simulink model "Non_Linear_Simulator_B747"  (R2020a)
settings: Solver=ode4  StartTime=0.0  StopTime=200  FixedStep=0.01  RelTol=1e-3
libraries: simulink_extras x7, shared6dof x1, vrlib x1
settings Model: OrderedModelArguments=off  Creator=mohan  LastModifiedBy=mohan

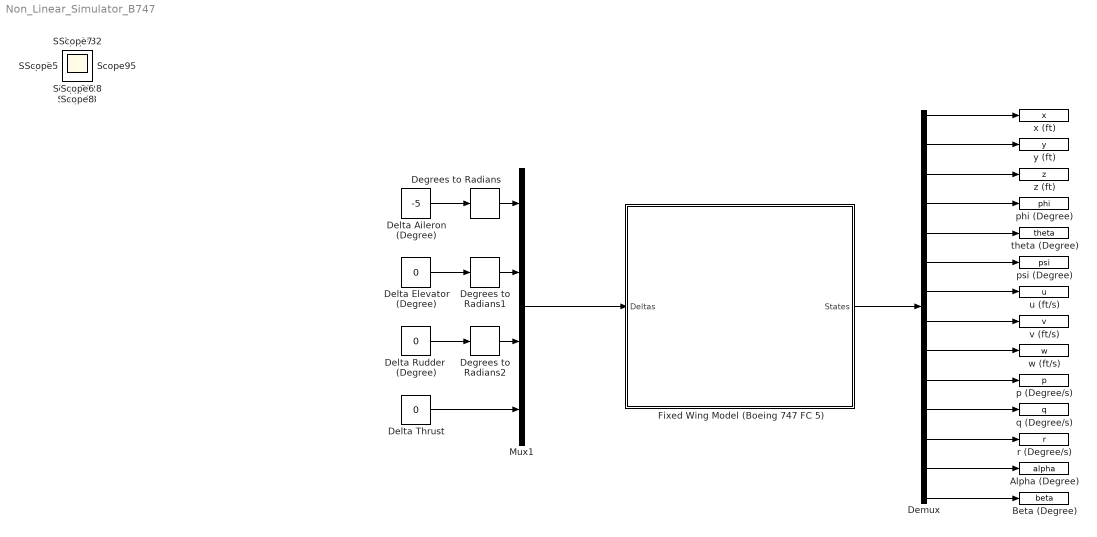
== system Non_Linear_Simulator_B747 ==
  Alpha (Degree) : ToWorkspace  VariableName=alpha  SaveFormat=Timeseries  SampleTime=-1
  Beta (Degree) : ToWorkspace  VariableName=beta  SaveFormat=Timeseries  SampleTime=-1
  Degrees to Radians : simulink_extras/Transformations/Degrees to Radians
  Degrees to Radians1 : simulink_extras/Transformations/Degrees to Radians
  Degrees to Radians2 : simulink_extras/Transformations/Degrees to Radians
  Delta Aileron (Degree) : Constant  Value=-5
  Delta Elevator (Degree) : Constant  Value=0
  Delta Rudder  (Degree) : Constant  Value=0
  Delta Thrust : Constant  Value=0
  Demux : Demux  Outputs=14
  Fixed Wing Model (Boeing 747 FC 5) : Subsystem  mask{m=19787.25091, g=32.17405, Ixx=1.82E+07, Iyy=3.31E+07, Izz=4.97E+07, Ixz=9.70E+05, Ixy=0, Iyz=0, L_th=1, VT=518, t0=0, tf=200, h=0.01, Xu=-0.00247, Zu=-0.0679, Mu=0.000247, Xw=0.0782, Zw=-0.433, Mw=-0.00170, Zw_dot=0.0157, Zq=-6.39, Mw_dot=-0.000125, Mq=-0.0421, Xdel_e=2.02, Zdel_e=-16.9, Mdel_e=-1.09, Xdel_t=0.505e-4, Zdel_t=-0.220e-5, Mdel_t=0.302e-6, Yv=-0.0822, YB=-42.6, LB_dash=-2.05, NB_dash=0.419, Lp_dash=-0.652, Np_dash=-0.0701, Lr_dash=0.376, Nr_dash=-0.140, Ydel_a_star=0, Ldel_a_dash=0.128, Ndel_a_dash=0.0177, Ydel_r_star=0.0131, Ldel_r_dash=0.148, Ndel_r_dash=-0.381, Yp=0, Yr=0, x0=0, y0=0, z0=-20000, u_0=514.3561332, v_0=0, w_0=61.33325558, p_0=0, q_0=0, r_0=0, udot_0=0, vdot_0=0, wdot_0=0, phai_0=0, theta_0=6.8*pi/180, psi_0=0}
      mask prompts: m "Mass"; g "Gravity"; L_th "Perpindicular Distance to Thrust Line from C.G"; VT "True Speed (FPS)"; t0 "Start Time"; tf "Stop Time"; h "Time Step"
      mask DialogControl Time Prompt: Time Properties
      mask DialogControl Derivatives Prompt: Aerodynamics Derivatives
      mask DialogControl States Prompt: Initial States
      mask Display: image('$imagefile'); % Use "Edit Image" on toolstrip to change.
  Mux1 : Mux
  p (Degree/s) : ToWorkspace  VariableName=p  SaveFormat=Timeseries  SampleTime=-1
  phi (Degree) : ToWorkspace  VariableName=phi  SaveFormat=Timeseries  SampleTime=-1
  psi (Degree) : ToWorkspace  VariableName=psi  SaveFormat=Timeseries  SampleTime=-1
  q (Degree/s) : ToWorkspace  VariableName=q  SaveFormat=Timeseries  SampleTime=-1
  r (Degree/s) : ToWorkspace  VariableName=r  SaveFormat=Timeseries  SampleTime=-1
  theta (Degree) : ToWorkspace  VariableName=theta  SaveFormat=Timeseries  SampleTime=-1
  u (ft/s) : ToWorkspace  VariableName=u  SaveFormat=Timeseries  SampleTime=-1
  v (ft/s) : ToWorkspace  VariableName=v  SaveFormat=Timeseries  SampleTime=-1
  w (ft/s) : ToWorkspace  VariableName=w  SaveFormat=Timeseries  SampleTime=-1
  x (ft) : ToWorkspace  VariableName=x  SaveFormat=Timeseries  SampleTime=-1
  y (ft) : ToWorkspace  VariableName=y  SaveFormat=Timeseries  SampleTime=-1
  z (ft) : ToWorkspace  VariableName=z  SaveFormat=Timeseries  SampleTime=-1
  Scope{,1..33} (34 alike) : Scope
  wires:
  Delta Elevator (Degree)/1 -> Degrees to Radians1/1
  Delta Thrust/1 -> Mux1/4
  Delta Aileron (Degree)/1 -> Degrees to Radians/1
  Delta Rudder  (Degree)/1 -> Degrees to Radians2/1
  Mux1/1 -> Fixed Wing Model (Boeing 747 FC 5)/1(Deltas)
  Fixed Wing Model (Boeing 747 FC 5)/1(States) -> Demux/1
  Demux/1 -> x (ft)/1
  Demux/2 -> y (ft)/1
  Demux/3 -> z (ft)/1
  Demux/5 -> theta (Degree)/1
  Demux/7 -> u (ft/s)/1
  Demux/8 -> v (ft/s)/1
  Demux/9 -> w (ft/s)/1
  Demux/10 -> p (Degree/s)/1
  Demux/11 -> q (Degree/s)/1
  Demux/12 -> r (Degree/s)/1
  Demux/13 -> Alpha (Degree)/1
  Demux/14 -> Beta (Degree)/1
  Degrees to Radians/1 -> Mux1/1
  Degrees to Radians1/1 -> Mux1/2
  Degrees to Radians2/1 -> Mux1/3
  Demux/4 -> phi (Degree)/1
  Demux/6 -> psi (Degree)/1

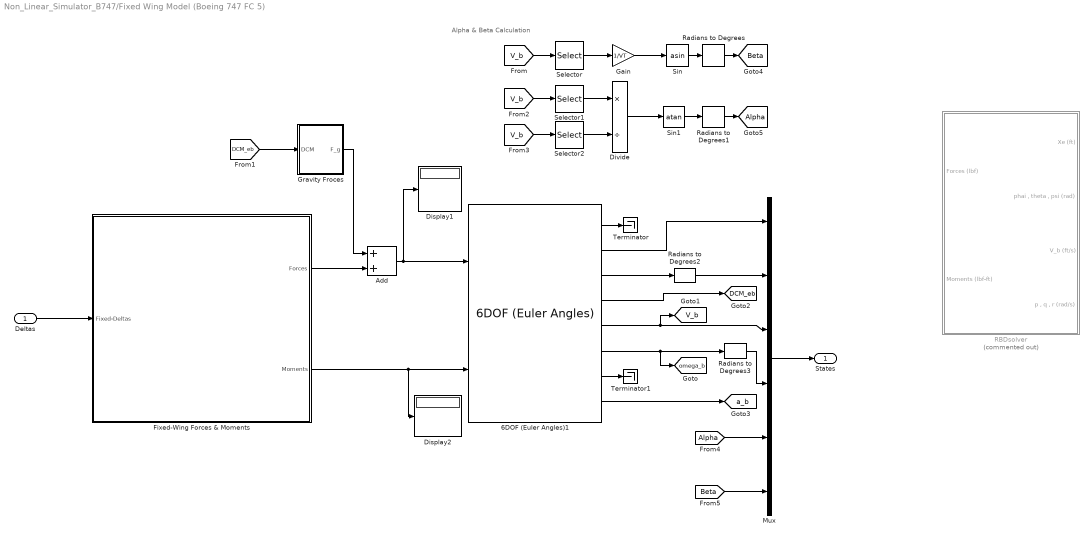
== system Non_Linear_Simulator_B747/Fixed Wing Model (Boeing 747 FC 5) ==
  note: Alpha & Beta Calculation
  Deltas : Inport
  6DOF (Euler Angles)1 : shared6dof/6DOF (Euler Angles)  units=English (Velocity in ft/s)  mtype=Fixed  rep=Euler Angles  xme_0=[x0 y0 z0]  Vm_0=[u_0 v_0 w_0]  eul_0=[phai_0 theta_0 psi_0]  pm_0=[p_0 q_0 r_0]  mass_0=m  mass_e=0.5  mass_f=2.0  inertia=[Ixx -Ixy -Ixz ; -Ixy Iyy -Iyz ; -Ixz -Iyz Izz]  inertia_e=eye(3)  inertia_f=2*eye(3)  k_quat=1.0  vre_flag=on  abi_flag=off  aMode=aMode  xme_statename=''  Vm_statename=''  eul_statename=''  quat_statename=''  pm_statename=''  mass_statename=''
      settings: SourceProductBaseCode=AE,PW,MT,VE,VP
  Add : Sum  Inputs=2
  Display1 : Display
  Display2 : Display
  Divide : Product  Inputs=*/
  Fixed-Wing Forces & Moments : Subsystem
  Gain : Gain  Gain=1/VT
  Gravity Froces : Subsystem
  Mux : Mux  Inputs=6
  RBDsolver : Subsystem  Commented=on
  Radians to Degrees{,1..3} (4 alike) : simulink_extras/Transformations/Radians to Degrees
  Selector : Selector  InputPortWidth=3  IndexOptions=Starting index (dialog)  Indices=2  OutputSizes=1
  Selector1 : Selector  InputPortWidth=3  IndexOptions=Starting index (dialog)  Indices=3  OutputSizes=1
  Selector2 : Selector  InputPortWidth=3  IndexOptions=Starting index (dialog)  Indices=1  OutputSizes=1
  Sin : Trigonometry  Operator=asin
  Sin1 : Trigonometry  Operator=atan
  Terminator : Terminator
  Terminator1 : Terminator
  States : Outport
  tag scope: Alpha=global, Beta=global, DCM_eb=global, V_b=global, a_b=global, omega_b=global
  wires:
  Gravity Froces/1(F_g) -> Add/1
  6DOF (Euler Angles)1/2 -> Mux/1
  6DOF (Euler Angles)1/1 -> Terminator/1
  Mux/1 -> States/1
  6DOF (Euler Angles)1/7 -> Terminator1/1
  Fixed-Wing Forces & Moments/1(Forces) -> Add/2
  Add/1 -> 6DOF (Euler Angles)1/1, Display1/1
  Fixed-Wing Forces & Moments/2("Moments ") -> Display2/1, 6DOF (Euler Angles)1/2
  6DOF (Euler Angles)1/4 -> [DCM_eb]
  6DOF (Euler Angles)1/8 -> [a_b]
  [DCM_eb] -> Gravity Froces/1(DCM)
  [V_b] -> Selector/1
  Selector/1 -> Gain/1
  Gain/1 -> Sin/1
  Sin/1 -> Radians to Degrees/1
  Divide/1 -> Sin1/1
  Selector1/1 -> Divide/1
  Sin1/1 -> Radians to Degrees1/1
  [V_b] -> Selector1/1
  [V_b] -> Selector2/1
  Selector2/1 -> Divide/2
  [Alpha] -> Mux/5
  [Beta] -> Mux/6
  Radians to Degrees/1 -> [Beta]
  Radians to Degrees1/1 -> [Alpha]
  6DOF (Euler Angles)1/3 -> Radians to Degrees2/1
  6DOF (Euler Angles)1/6 -> [omega_b], Radians to Degrees3/1
  Deltas/1 -> Fixed-Wing Forces & Moments/1(Fixed-Deltas)
  Radians to Degrees2/1 -> Mux/2
  6DOF (Euler Angles)1/5 -> Mux/3, [V_b]
  Radians to Degrees3/1 -> Mux/4

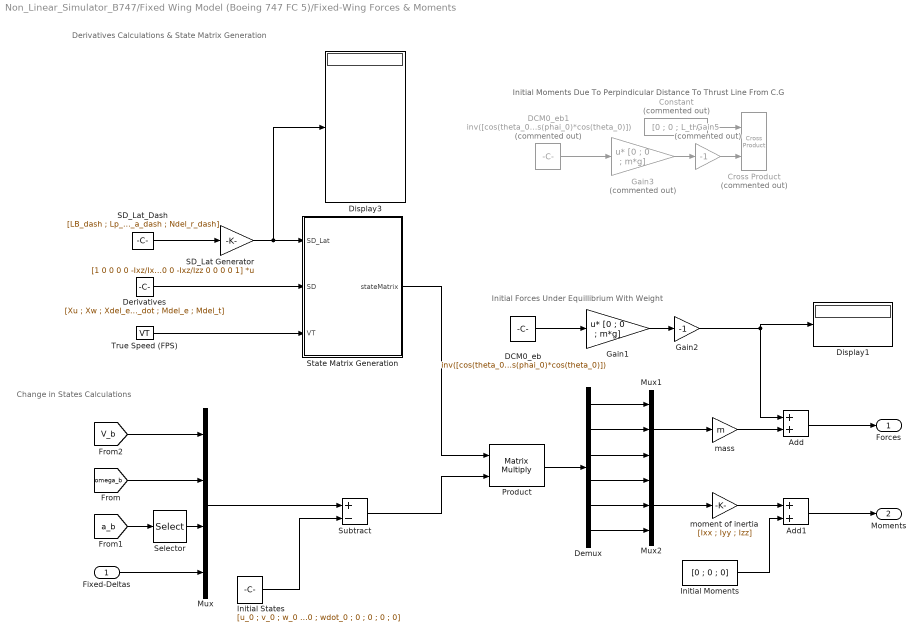
== system Non_Linear_Simulator_B747/Fixed Wing Model (Boeing 747 FC 5)/Fixed-Wing Forces & Moments ==
  note: Change in States Calculations
  note: Derivatives Calculations & State Matrix Generation
  note: Initial Forces Under Equillibrium With Weight
  note: Initial Moments Due To Perpindicular Distance To Thrust Line From C.G
  Fixed-Deltas : Inport
  Add : Sum
  Add1 : Sum
  Constant : Constant  Commented=on  Value=[0 ; 0 ; L_th]
  Cross Product : vrlib/Utilities/Cross Product  Commented=on
  DCM0_eb : Constant  Value="inv([cos(theta_0)*cos(psi_0) , (sin(phai_0)*sin(theta_0)*cos(psi_0)-cos(phai_0)*sin(psi_0)) , (cos(phai_0)*sin(theta_0)*cos(psi_0)+sin(phai_0)*sin(psi_0)) ; cos(theta_0)*sin(psi_0) , (sin(phai_0)*sin(theta_0)*sin(psi_0)+cos(phai_0)*cos(psi_0)) , (cos(phai_0)*sin(theta_0)*sin(psi_0)-sin(phai_0)*cos(psi_0)) ;  -sin(theta_0) ,  sin(phai_0)*cos(theta_0)  , cos(phai_0)*cos(theta_0)])"
  DCM0_eb1 : Constant  Commented=on  Value="inv([cos(theta_0)*cos(psi_0) , (sin(phai_0)*sin(theta_0)*cos(psi_0)-cos(phai_0)*sin(psi_0)) , (cos(phai_0)*sin(theta_0)*cos(psi_0)+sin(phai_0)*sin(psi_0)) ; cos(theta_0)*sin(psi_0) , (sin(phai_0)*sin(theta_0)*sin(psi_0)+cos(phai_0)*cos(psi_0)) , (cos(phai_0)*sin(theta_0)*sin(psi_0)-sin(phai_0)*cos(psi_0)) ;  -sin(theta_0) ,  sin(phai_0)*cos(theta_0)  , cos(phai_0)*cos(theta_0)])"
  Demux : Demux  Outputs=6
  Derivatives : Constant  Value=[Xu ; Xw ; Xdel_e ; Xdel_t ; Yv ; Yp ; Yr ; Ydel_r_star ; Zu ; Zw ; Zq ; Zw_dot ; Zdel_e ; Zdel_t ; Mu ; Mw ; Mq ; Mw_dot ; Mdel_e ; Mdel_t]
  Display1 : Display
      settings: Decimation=4
  Display3 : Display
  Gain1 : Gain  Gain=[0 ; 0 ; m*g]  Multiplication=Matrix(u*K)
  Gain2 : Gain  Gain=-1
  Gain3 : Gain  Commented=on  Gain=[0 ; 0 ; m*g]  Multiplication=Matrix(u*K)
  Gain5 : Gain  Commented=on  Gain=-1
  Initial Moments : Constant  Value=[0 ; 0 ; 0]
  Initial States : Constant  Value=[u_0 ; v_0 ; w_0 ; p_0 ; q_0 ; r_0 ; wdot_0 ; 0 ; 0 ; 0 ; 0]
  Mux : Mux
  Mux1 : Mux  Inputs=3
  Mux2 : Mux  Inputs=3
  Product : Product  Multiplication=Matrix(*)
  SD_Lat Generator : Gain  Gain="[1 0 0 0 0 -Ixz/Ixx 0 0 0 0 ; 0 1 0 0 0 0 -Ixz/Ixx 0 0 0 ; 0 0 1 0 0 0 0 -Ixz/Ixx 0  0 ; 0 0 0 1 0 0 0 0 -Ixz/Ixx 0 ; 0 0 0 0 1 0 0 0 0 -Ixz/Ixx ; -Ixz/Izz 0 0 0 0 1 0 0 0 0 ; 0 -Ixz/Izz 0 0 0 0 1 0 0 0 ; 0 0 -Ixz/Izz 0 0 0 0 1 0 0 ; 0 0 0 -Ixz/Izz 0 0 0 0 1 0 ;  0 0 0 0 -Ixz/Izz 0 0 0 0 1]"  Multiplication=Matrix(K*u)
  SD_Lat_Dash : Constant  Value=[LB_dash ; Lp_dash ; Lr_dash ; Ldel_a_dash ; Ldel_r_dash ; NB_dash ; Np_dash ; Nr_dash ; Ndel_a_dash ; Ndel_r_dash]
  Selector : Selector  InputPortWidth=3  IndexOptions=Starting index (dialog)  Indices=3  OutputSizes=1
  State Matrix Generation : MATLAB Function  TreatAsAtomicUnit=on
  Subtract : Sum  Inputs=+-
  True Speed (FPS) : Constant  Value=VT
  mass : Gain  Gain=m
  moment of inertia : Gain  Gain=[Ixx ; Iyy ; Izz]
  Forces : Outport
  "Moments " : Outport  Port=2
  wires:
  Selector/1 -> Mux/3
  Fixed-Deltas/1 -> Mux/4
  [omega_b] -> Mux/2
  [V_b] -> Mux/1
  Mux/1 -> Subtract/1
  Subtract/1 -> Product/2
  Initial States/1 -> Subtract/2
  Demux/2 -> Mux1/2
  Demux/1 -> Mux1/1
  Demux/3 -> Mux1/3
  Demux/4 -> Mux2/1
  Demux/5 -> Mux2/2
  Demux/6 -> Mux2/3
  Mux1/1 -> mass/1
  Mux2/1 -> moment of inertia/1
  mass/1 -> Add/2
  moment of inertia/1 -> Add1/1
  Add/1 -> Forces/1
  Add1/1 -> "Moments "/1
  DCM0_eb/1 -> Gain1/1
  Gain1/1 -> Gain2/1
  Gain2/1 -> Add/1, Display1/1
  Gain3/1 -> Gain5/1
  DCM0_eb1/1 -> Gain3/1
  Gain5/1 -> Cross Product/2
  Constant/1 -> Cross Product/1
  Initial Moments/1 -> Add1/2
  SD_Lat_Dash/1 -> SD_Lat Generator/1
  SD_Lat Generator/1 -> Display3/1, State Matrix Generation/1(SD_Lat)
  Product/1 -> Demux/1
  State Matrix Generation/1(stateMatrix) -> Product/1
  Derivatives/1 -> State Matrix Generation/2(SD)
  True Speed (FPS)/1 -> State Matrix Generation/3(VT)
  [a_b] -> Selector/1

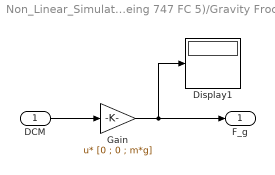
== system Non_Linear_Simulator_B747/Fixed Wing Model (Boeing 747 FC 5)/Gravity Froces ==
  DCM : Inport
  Display1 : Display
  Gain : Gain  Gain=[0 ; 0 ; m*g]  Multiplication=Matrix(u*K)
  F_g : Outport
  wires:
  Gain/1 -> F_g/1, Display1/1
  DCM/1 -> Gain/1

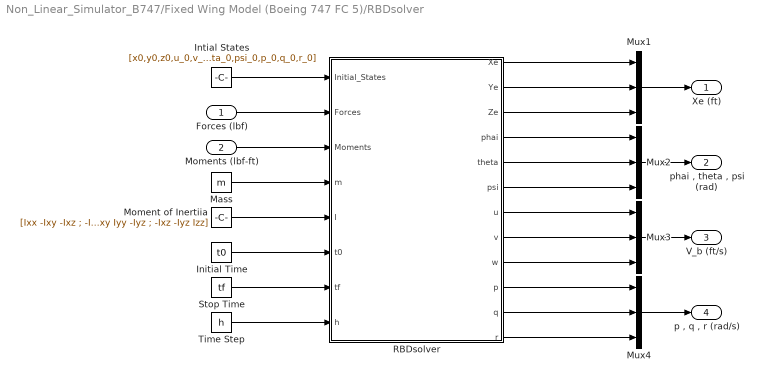
== system Non_Linear_Simulator_B747/Fixed Wing Model (Boeing 747 FC 5)/RBDsolver ==
  Forces (lbf) : Inport
  Moments (lbf-ft) : Inport  Port=2
  Initial Time : Constant  Value=t0
  Intial States : Constant  Value=[x0,y0,z0,u_0,v_0,w_0,phai_0,theta_0,psi_0,p_0,q_0,r_0]
  Mass : Constant  Value=m
  Moment of Inertiia : Constant  Value=[Ixx -Ixy -Ixz ; -Ixy Iyy -Iyz ; -Ixz -Iyz Izz]
  Mux{1..4} (4 alike) : Mux  Inputs=3
  RBDsolver : MATLAB Function  TreatAsAtomicUnit=on
  Stop Time : Constant  Value=tf
  Time Step : Constant  Value=h
  Xe (ft) : Outport
  "phai , theta , psi (rad)" : Outport  Port=2
  V_b (ft/s) : Outport  Port=3
  "p , q , r (rad/s)" : Outport  Port=4
  wires:
  RBDsolver/5(theta) -> Mux2/2
  Intial States/1 -> RBDsolver/1(Initial_States)
  Forces (lbf)/1 -> RBDsolver/2(Forces)
  RBDsolver/11(q) -> Mux4/2
  RBDsolver/7(u) -> Mux3/1
  RBDsolver/8(v) -> Mux3/2
  RBDsolver/9(w) -> Mux3/3
  Mass/1 -> RBDsolver/4(m)
  Moments (lbf-ft)/1 -> RBDsolver/3(Moments)
  Stop Time/1 -> RBDsolver/7(tf)
  Initial Time/1 -> RBDsolver/6(t0)
  RBDsolver/10(p) -> Mux4/1
  Time Step/1 -> RBDsolver/8(h)
  Moment of Inertiia/1 -> RBDsolver/5(I)
  RBDsolver/6(psi) -> Mux2/3
  RBDsolver/4(phai) -> Mux2/1
  RBDsolver/1(Xe) -> Mux1/1
  RBDsolver/3(Ze) -> Mux1/3
  RBDsolver/2(Ye) -> Mux1/2
  RBDsolver/12(r) -> Mux4/3
  Mux1/1 -> Xe (ft)/1
  Mux2/1 -> "phai , theta , psi (rad)"/1
  Mux3/1 -> V_b (ft/s)/1
  Mux4/1 -> "p , q , r (rad/s)"/1

== matlab function Non_Linear_Simulator_B747/Fixed Wing Model (Boeing 747 FC 5)/Fixed-Wing Forces & Moments/State Matrix Generation ==
  data: SD_Lat input; stateMatrix output; SD input; VT input
function stateMatrix = stateMatrixGenerator(SD_Lat,SD,VT)
stateMatrix=zeros(6,11);

Xu=SD(1);   Xw=SD(2);       Xdel_e=SD(3);       Xdel_t=SD(4);   Yv=SD(5);
Yp=SD(6);   Yr=SD(7);       Ydel_r_star=SD(8);  Zu=SD(9);       Zw=SD(10);
Zq=SD(11);  Zw_dot=SD(12);  Zdel_e=SD(13);      Zdel_t=SD(14);   Mu=SD(15); 
Mw=SD(16);  Mq=SD(17);      Mw_dot=SD(18);      Mdel_e=SD(19);   Mdel_t=SD(20);

LB=SD_Lat(1);   Lp=SD_Lat(2);   Lr=SD_Lat(3);   Ldel_a=SD_Lat(4);
Ldel_r=SD_Lat(5);
NB=SD_Lat(6);   Np=SD_Lat(7);   Nr=SD_Lat(8);   Ndel_a=SD_Lat(9);   
Ndel_r=SD_Lat(10);

Ydel_r=Ydel_r_star*VT;
Lv=LB/VT;
Nv=NB/VT;

stateMatrix=...
     [Xu , 0 , Xw , 0 , 0 , 0 , 0 , 0 , Xdel_e , 0 , Xdel_t ; 
      0 , Yv , 0 , Yp , 0 , Yr , 0 , 0 , 0 , Ydel_r , 0 ; 
      Zu , 0 , Zw , 0 , Zq , 0 , Zw_dot , 0 , Zdel_e , 0 , Zdel_t ; 
      0 , Lv , 0 , Lp , 0 , Lr , 0 , Ldel_a , 0 , Ldel_r , 0 ; 
      Mu , 0 , Mw , 0 , Mq , 0 , Mw_dot , 0 , Mdel_e , 0 , Mdel_t ; 
      0 , Nv , 0 , Np , 0 , Nr , 0 , Ndel_a , 0 , Ndel_r , 0];
end

== matlab function Non_Linear_Simulator_B747/Fixed Wing Model (Boeing 747 FC 5)/RBDsolver/RBDsolver ==
  data: Initial_States input; Xe output; Forces input; Moments input; m input; I input; t0 input; tf input; h input; Ye output; Ze output; phai output; theta output; psi output; u output; v output; w output; p output; q output; r output
function [Xe,Ye,Ze,phai,theta,psi,u,v,w,p,q,r] = RBDsolver(Initial_States,Forces,Moments,m,I,t0,tf,h)
    tspan=t0:h:tf;
    states_final=zeros(length(tspan),12);
    states_final(1,:)=Initial_States;
    K=zeros(4,12);
    for i=1:(length(tspan)-1)
        K(1,:)=(h*feval(@odefunc,states_final(i,:)'))';
        K(2,:)=(h*feval(@odefunc,(states_final(i,:)'+0.5*K(1,:)')))'; 
        K(3,:)=(h*feval(@odefunc,(states_final(i,:)'+0.5*K(2,:)')))';
        K(4,:)=(h*feval(@odefunc,(states_final(i,:)'+K(3,:)')))';    
        states_final(i+1,:)=states_final(i,:)+(1/6)*(K(1,:)+2*K(2,:)+2*K(3,:)+K(4,:));
        % Euler Angles must be bounded by pi , -pi
        if (states_final(i+1,7)>=pi)
            states_final(i+1,7)=states_final(i+1,7)-2*pi;
        elseif (states_final(i+1,7)<=-pi)
            states_final(i+1,7)=states_final(i+1,7)+2*pi;
        elseif (states_final(i+1,8)>=pi)
            states_final(i+1,8)=states_final(i+1,8)-2*pi;
        elseif (states_final(i+1,8)<=-pi)
            states_final(i+1,8)=states_final(i+1,8)+2*pi;
        elseif (states_final(i+1,9)>=pi)
            states_final(i+1,9)=states_final(i+1,9)-2*pi;
        elseif (states_final(i+1,9)<=-pi)
            states_final(i+1,9)=states_final(i+1,9)+2*pi;
        end
    end
    Xe=states_final(:,1);
    Ye=states_final(:,2);
    Ze=states_final(:,3);
    u=states_final(:,4);
    v=states_final(:,5);
    w=states_final(:,6);
    phai=states_final(:,7);
    theta=states_final(:,8);
    psi=states_final(:,9);
    p=states_final(:,10);
    q=states_final(:,11);
    r=states_final(:,12);

    function [dstates_dt] = odefunc(states)
        DCM_be=[cos(states(8))*cos(states(9)) , (sin(states(7))*sin(states(8))*cos(states(9))-cos(states(7))*sin(states(9))) , (cos(states(7))*sin(states(8))*cos(states(9))+sin(states(7))*sin(states(9)));
             cos(states(8))*sin(states(9)) , (sin(states(7))*sin(states(8))*sin(states(9))+cos(states(7))*cos(states(9))) , (cos(states(7))*sin(states(8))*sin(states(9))-sin(states(7))*cos(states(9)));
             -sin(states(8))               ,  sin(states(7))*cos(states(8))                                               , cos(states(7))*cos(states(8))];

        Euler_Matrix=[1 ,  sin(states(7))*tan(states(8))   ,    cos(states(7))*tan(states(8));
                      0 ,  cos(states(7))                  ,   -sin(states(7)); 
                      0 ,  sin(states(7))/cos(states(8))   ,   cos(states(7))/cos(states(8))];
        
        Gravity_e=[0;0;m*9.807];
        
        Forces_tot=Forces+inv(DCM_be)*Gravity_e;

        dposition_dt=DCM_be*[states(4) ; states(5) ; states(6)];

        dvelocity_dt=Forces_tot./m-((cross([states(10),states(11),states(12)],[states(4),states(5),states(6)]))');

        dorientation_dt=Euler_Matrix*[states(10) ; states(11) ; states(12)];

        dpqr_dt=inv(I)*(Moments-cross([states(10) ; states(11) ; states(12)],(I*[states(10) ; states(11) ; states(12)])));

        dstates_dt=[dposition_dt ; dvelocity_dt ; dorientation_dt ; dpqr_dt];
    end               
end
